simulink library "DelayLibraryRmdl"  (R2022b)
settings: Solver=VariableStepAuto  StartTime=0.0  StopTime=10.0  RelTol=1e-3
undefined symbols (not defined in the file or in its folder): delay_chain, Generic, L, max_delay, num_input_chs, Row
libraries: AudioStats x4, FeaturePath x3, TuneVar x3, TOP x1, RTC x1, $bdroot x1
(part 2 of 2)

== matlab function DelayLibraryRmdl/PoolDelay/pool delay init ==
  data: u input; delayChain input; codeWorkMemory data_store_memory; variantSelect parameter; delayBuffer data_store_memory; fastDelayBuffer data_store_memory; RMDLshutdown data_store_memory
  events: trigger input FUNCTION_CALL_EVENT
function pool_delay_init(u, delayChain, variantSelect)

% Pool delay function provides delay lines for N channels.  Core
% implementation provides delay of any positive integer value.  MDMA
% implementation provides integer value delays of a frame or greater. 
% 
% Parameters:
%   u:              Input channels [frame size x number of inputs]
%   delayChain:     Delay in samples for each channel [1 x delay per channel]
%   variantSelect:  Variant selection of implementation (scaler)
%
% Global parameters:
%   delayBuffer:    Delay line circular buffer containing all channel  
%                   delay state data
%   fastDelayBuffer: Fast delay line circular buffer containing all channel  
%                    delay state data
%   codeWorkMemory: Working memory set up during roommode reset/init CRL
%                   function call [1 x codeWorkMemorySize]
%   RMDLshutdown: Flag to indicate RMDL is in progress [1 x 1]

% Extract configuration information from inut
[frameSize, numChannels]  = size(u);

global delayBuffer;
global fastDelayBuffer;
global codeWorkMemory;
global RMDLshutdown;

% Get the work memory and delay buffer sizes
workMemorySize = numel(codeWorkMemory);
delayBufferSize = numel(delayBuffer);
fastDelayBufferSize = numel(fastDelayBuffer);

% Set correct data types
frameSize = uint32(frameSize);
numChannels = uint32(numChannels);
delayChain = uint32(delayChain);
workMemorySize = uint32(workMemorySize);
delayBufferSize = uint32(delayBufferSize);
fastDelayBufferSize = uint32(fastDelayBufferSize);
    
% There are three implementation types:
% Type       Value     Description
% L1 Memory    1       Optimized CRL C code using L1 memory delay buffer and 
%                      core for movement of data in/out of delay buffer
% L2 Memory    2       Optimized CRL C code using L2 memory delay buffer and
%                      MDMA for movement of data in/out of delay buffer
% Generic      3       Generic implementation for other targets without CRL 
%
% NOTE: Generic implementation does not use codeWorkMemory, thus does not
% need any custom initialization.
if (variantSelect == 1)
    y = pool_delay_core_init(u, fastDelayBuffer, fastDelayBufferSize, ...
                             delayChain, numChannels, frameSize, ...
                             codeWorkMemory, workMemorySize);

                         
    % NOTE: The CRL mechanism requires an output for the function call,
    % and appears to be optimized out if that return value isn't used. 
    % This is a dummy operation to make sure CRL ends up in generated code
    codeWorkMemory(1) = y; 
elseif (variantSelect == 2)
    y = pool_delay_mdma_init(u, delayBuffer, delayBufferSize, ...
                             fastDelayBuffer, fastDelayBufferSize, ...
                             delayChain, numChannels, frameSize, ...
                             codeWorkMemory, workMemorySize);
    
    % NOTE: The CRL mechanism requires an output for the function call,
    % and appears to be optimized out if that return value isn't used. 
    % This is a dummy operation to make sure CRL ends up in generated code
    codeWorkMemory(1) = y; 
end

% Set flag to indicate initialization has completed and step functions can
% start running.
RMDLshutdown = uint32(1);

end


% Pool delay CRL core initialization function conceptual specification  
function y = pool_delay_core_init(u, fastDelayBuffer, fastDelayBufferSize, ... 
                                  delayChain, numChannels, frameSize, ...
                                  workMemory, workMemorySize)
% If target == codegen, error out if no CRL found
coder.replace('-errorifnoreplacement');

% No init simulation code, but need to do something to ensure CRL does not
% get optimized out
y = single(workMemory(1) + 1);

end


% Pool delay CRL MDMA initialization function conceptual specification
function y = pool_delay_mdma_init(u, delayBuffer, delayBufferSize, ...
                                  fastDelayBuffer, fastDelayBufferSize, ...
                                  delayChain, numChannels, frameSize, ...
                                  workMemory, workMemorySize) 
% If target == codegen, error out if no CRL found
coder.replace('-errorifnoreplacement');

% No init simulation code, but need to do something to ensure CRL does not
% get optimized out
y = single(workMemory(1) + 1);

end

== matlab function DelayLibraryRmdl/PoolDelay/ITC/init ==
  events: trigger input FUNCTION_CALL_EVENT; init output FUNCTION_CALL_EVENT
function init
% Call the init function
init();
